simulink library "amg_high_precision_rtc"  (R2015b)
settings: Solver=ode45  StartTime=0.0  StopTime=10.0  RelTol=1e-3
libraries: simulink x207, waijung_soft_i2c_lib x11, amg_high_precision_rtc x10
(part 4 of 5)

== system amg_high_precision_rtc/Soft I2C/Soft-DS3231 Configure/Enabled Subsystem/Debouce2/Enabled Subsystem1 ==
  Enable : EnablePort  PropagateVarSize=During execution
  Bitwise Operator : simulink/Logic and Bit Operations/Bitwise Operator  logicop=AND  UseBitMask=on  BitMask=1  BitMaskRealWorld=Stored Integer
  Compare To Zero : simulink/Logic and Bit Operations/Compare To Zero  SystemSampleTime=-1  relop===  LogicOutDataTypeMode=uint8  ZeroCross=off
  Counter Free-Running : simulink/Sources/Counter Free-Running  SystemSampleTime=-1  NumBits=32  tsamp=-1
  Out1 : Outport  InitialOutput=0
  wires:
  Compare To Zero/1 -> Out1/1
  Bitwise Operator/1 -> Compare To Zero/1
  Counter Free-Running/1 -> Bitwise Operator/1

== system amg_high_precision_rtc/Soft I2C/Soft-DS3231 Configure/Enabled Subsystem/Debouce2/Enabled Subsystem4 ==
  Enable : EnablePort  PropagateVarSize=During execution
  Counter Free-Running : simulink/Sources/Counter Free-Running  SystemSampleTime=-1  NumBits=32  tsamp=-1
  Out1 : Outport  InitialOutput=0
  wires:
  Counter Free-Running/1 -> Out1/1

== system amg_high_precision_rtc/Soft I2C/Soft-DS3231 Configure/Enabled Subsystem/Debouce2/Enabled Subsystem5 ==
  Enable : EnablePort  PropagateVarSize=During execution
  Counter Free-Running : simulink/Sources/Counter Free-Running  SystemSampleTime=-1  NumBits=32  tsamp=-1
  Out1 : Outport  InitialOutput=0
  wires:
  Counter Free-Running/1 -> Out1/1

== system amg_high_precision_rtc/Soft I2C/Soft-DS3231 Configure/Enabled Subsystem/Debouce3/Enabled Subsystem ==
  Enable : EnablePort  PropagateVarSize=During execution
  Counter Free-Running : simulink/Sources/Counter Free-Running  SystemSampleTime=-1  NumBits=32  tsamp=-1
  Out1 : Outport  InitialOutput=0
  wires:
  Counter Free-Running/1 -> Out1/1

== system amg_high_precision_rtc/Soft I2C/Soft-DS3231 Configure/Enabled Subsystem/Debouce3/Enabled Subsystem1 ==
  Enable : EnablePort  PropagateVarSize=During execution
  Bitwise Operator : simulink/Logic and Bit Operations/Bitwise Operator  logicop=AND  UseBitMask=on  BitMask=1  BitMaskRealWorld=Stored Integer
  Compare To Zero : simulink/Logic and Bit Operations/Compare To Zero  SystemSampleTime=-1  relop===  LogicOutDataTypeMode=uint8  ZeroCross=off
  Counter Free-Running : simulink/Sources/Counter Free-Running  SystemSampleTime=-1  NumBits=32  tsamp=-1
  Out1 : Outport  InitialOutput=0
  wires:
  Compare To Zero/1 -> Out1/1
  Bitwise Operator/1 -> Compare To Zero/1
  Counter Free-Running/1 -> Bitwise Operator/1

== system amg_high_precision_rtc/Soft I2C/Soft-DS3231 Configure/Enabled Subsystem/Debouce3/Enabled Subsystem4 ==
  Enable : EnablePort  PropagateVarSize=During execution
  Counter Free-Running : simulink/Sources/Counter Free-Running  SystemSampleTime=-1  NumBits=32  tsamp=-1
  Out1 : Outport  InitialOutput=0
  wires:
  Counter Free-Running/1 -> Out1/1

== system amg_high_precision_rtc/Soft I2C/Soft-DS3231 Configure/Enabled Subsystem/Debouce3/Enabled Subsystem5 ==
  Enable : EnablePort  PropagateVarSize=During execution
  Counter Free-Running : simulink/Sources/Counter Free-Running  SystemSampleTime=-1  NumBits=32  tsamp=-1
  Out1 : Outport  InitialOutput=0
  wires:
  Counter Free-Running/1 -> Out1/1

== system amg_high_precision_rtc/Soft I2C/Soft-DS3231 Configure/Enabled Subsystem/Generate Mode ID/Enabled Subsystem2 ==
  Enable : EnablePort  PropagateVarSize=During execution
  Bitwise Operator : simulink/Logic and Bit Operations/Bitwise Operator  logicop=AND  UseBitMask=on  BitMask=7  BitMaskRealWorld=Stored Integer
  Counter Free-Running : simulink/Sources/Counter Free-Running  SystemSampleTime=-1  NumBits=16  tsamp=-1
  Out1 : Outport  InitialOutput=0
  wires:
  Bitwise Operator/1 -> Out1/1
  Counter Free-Running/1 -> Bitwise Operator/1

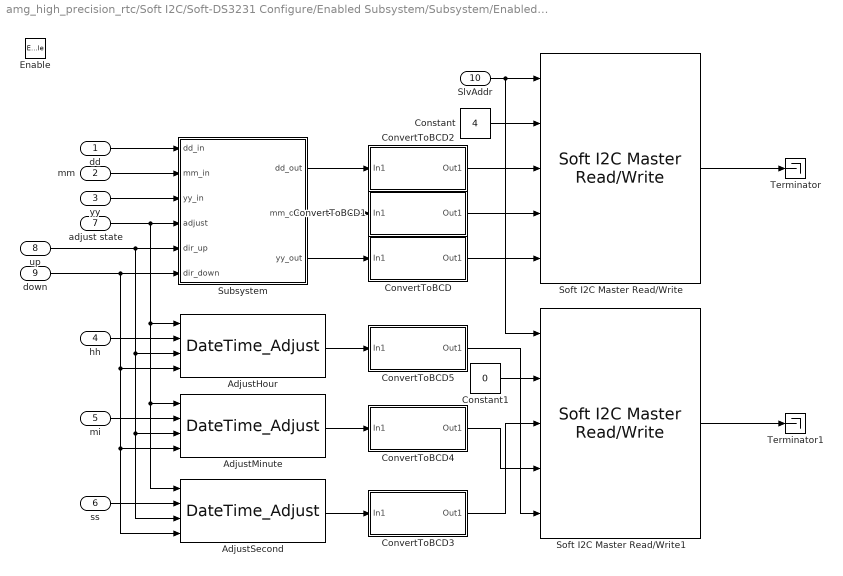
== system amg_high_precision_rtc/Soft I2C/Soft-DS3231 Configure/Enabled Subsystem/Subsystem/Enabled Subsystem ==
  dd : Inport
  mm : Inport  Port=2
  yy : Inport  Port=3
  hh : Inport  Port=4
  mi : Inport  Port=5
  ss : Inport  Port=6
  adjust state : Inport  Port=7
  up : Inport  Port=8
  down : Inport  Port=9
  SlvAddr : Inport  Port=10
  Enable : EnablePort  PropagateVarSize=During execution
  AdjustHour : amg_high_precision_rtc/DateTime_Adjust  SystemSampleTime=-1  state=3  max=23  min=0
  AdjustMinute : amg_high_precision_rtc/DateTime_Adjust  SystemSampleTime=-1  state=4  max=59  min=0
  AdjustSecond : amg_high_precision_rtc/DateTime_Adjust  SystemSampleTime=-1  state=5  max=59  min=0
  Constant : Constant  Value=4  OutDataTypeStr=uint8
  Constant1 : Constant  Value=0  OutDataTypeStr=uint8
  ConvertToBCD : Subsystem  TreatAsAtomicUnit=on
      settings: RTWFcnNameOpts=Use subsystem name  RTWFileNameOpts=Use function name
      mask Display: disp('Dec-to-BCD');
  ConvertToBCD1 : Subsystem  TreatAsAtomicUnit=on
      settings: RTWFcnNameOpts=Use subsystem name  RTWFileNameOpts=Use function name
      mask Display: disp('Dec-to-BCD');
  ConvertToBCD2 : Subsystem  TreatAsAtomicUnit=on
      settings: RTWFcnNameOpts=Use subsystem name  RTWFileNameOpts=Use function name
      mask Display: disp('Dec-to-BCD');
  ConvertToBCD3 : Subsystem  TreatAsAtomicUnit=on
      settings: RTWFcnNameOpts=Use subsystem name  RTWFileNameOpts=Use function name
      mask Display: disp('Dec-to-BCD');
  ConvertToBCD4 : Subsystem  TreatAsAtomicUnit=on
      settings: RTWFcnNameOpts=Use subsystem name  RTWFileNameOpts=Use function name
      mask Display: disp('Dec-to-BCD');
  ConvertToBCD5 : Subsystem  TreatAsAtomicUnit=on
      settings: RTWFcnNameOpts=Use subsystem name  RTWFileNameOpts=Use function name
      mask Display: disp('Dec-to-BCD');
  Soft I2C Master Read/Write : waijung_soft_i2c_lib/Soft I2C Master Read//Write  conf=ReadWrite  targetname=0  module=1  transfer=Blocking  clk=100  timeout=25  sdapins={'A4','A6'}  sclpins='A5'  writecount=4  readcount=0  waittime=0  forcestop=off  portpinstr=0  sampletime=inf  blockid=SoftI2CSoftDS3231ConfigureEnabledSubsystemSubsystemEnabledSubsystemSoftI2CMasterReadWrite  inputporttype=[3 3 3 3 3]  inputportwidth=[]  inputportlabel={'SlvAddr' 'Wr0 (uint8)' 'Wr1 (uint8)' 'Wr2 (uint8)' 'Wr3 (uint8)'}  outputporttype=[3]  outputportwidth=[1]  outputportlabel={'Status'}  compat=0  optionstring=[]
  Soft I2C Master Read/Write1 : waijung_soft_i2c_lib/Soft I2C Master Read//Write  conf=ReadWrite  targetname=0  module=1  transfer=Blocking  clk=100  timeout=25  sdapins={'A4','A6'}  sclpins='A5'  writecount=4  readcount=0  waittime=0  forcestop=off  portpinstr=0  sampletime=inf  blockid=SoftI2CSoftDS3231ConfigureEnabledSubsystemSubsystemEnabledSubsystemSoftI2CMasterReadWrite  inputporttype=[3 3 3 3 3]  inputportwidth=[]  inputportlabel={'SlvAddr' 'Wr0 (uint8)' 'Wr1 (uint8)' 'Wr2 (uint8)' 'Wr3 (uint8)'}  outputporttype=[3]  outputportwidth=[1]  outputportlabel={'Status'}  compat=0  optionstring=[]
  Subsystem : Subsystem
  Terminator : Terminator
  Terminator1 : Terminator
  wires:
  ConvertToBCD3/1(Out1) -> Soft I2C Master Read/Write1/3
  ConvertToBCD5/1(Out1) -> Soft I2C Master Read/Write1/5
  AdjustSecond/1 -> ConvertToBCD3/1(In1)
  AdjustMinute/1 -> ConvertToBCD4/1(In1)
  AdjustHour/1 -> ConvertToBCD5/1(In1)
  ConvertToBCD4/1(Out1) -> Soft I2C Master Read/Write1/4
  Soft I2C Master Read/Write1/1 -> Terminator1/1
  Constant1/1 -> Soft I2C Master Read/Write1/2
  hh/1 -> AdjustHour/2
  mi/1 -> AdjustMinute/2
  ss/1 -> AdjustSecond/2
  ConvertToBCD/1(Out1) -> Soft I2C Master Read/Write/5
  ConvertToBCD1/1(Out1) -> Soft I2C Master Read/Write/4
  ConvertToBCD2/1(Out1) -> Soft I2C Master Read/Write/3
  Soft I2C Master Read/Write/1 -> Terminator/1
  Constant/1 -> Soft I2C Master Read/Write/2
  Subsystem/3(yy_out) -> ConvertToBCD/1(In1)
  Subsystem/2(mm_out) -> ConvertToBCD1/1(In1)
  Subsystem/1(dd_out) -> ConvertToBCD2/1(In1)
  SlvAddr/1 -> Soft I2C Master Read/Write/1, Soft I2C Master Read/Write1/1
  down/1 -> AdjustSecond/4, AdjustMinute/4, AdjustHour/4, Subsystem/6(dir_down)
  up/1 -> AdjustSecond/3, AdjustMinute/3, AdjustHour/3, Subsystem/5(dir_up)
  adjust state/1 -> AdjustSecond/1, AdjustMinute/1, AdjustHour/1, Subsystem/4(adjust)
  yy/1 -> Subsystem/3(yy_in)
  mm/1 -> Subsystem/2(mm_in)
  dd/1 -> Subsystem/1(dd_in)

== system amg_high_precision_rtc/Soft I2C/Soft-DS3231 Configure/Enabled Subsystem/Subsystem/Soft-DS3231 Get Date ==
  Slave Address : Inport
  Compare To Zero : simulink/Logic and Bit Operations/Compare To Zero  SystemSampleTime=-1  relop===  LogicOutDataTypeMode=uint8  ZeroCross=off
  Convert : Subsystem  TreatAsAtomicUnit=on
  REG_DATE : Constant  Value=hex2dec('03')  OutDataTypeStr=uint8
  Soft I2C Master Read/Write : waijung_soft_i2c_lib/Soft I2C Master Read//Write  conf=ReadWrite  targetname=0  module=1  transfer=Blocking  clk=100  timeout=25  sdapins={'A4','A6'}  sclpins='A5'  writecount=1  readcount=4  waittime=0  forcestop=off  portpinstr=0  sampletime=-1  blockid=SoftI2CSoftDS3231GetDateSoftI2CMasterReadWrite  inputporttype=[3 3]  inputportwidth=[]  inputportlabel={'SlvAddr' 'Wr0 (uint8)'}  outputporttype="[3 3 3 3 3    ]"  outputportwidth=[1 1 1 1 1]  outputportlabel={'Status' 'Rd0 (uint8)' 'Rd1 (uint8)' 'Rd2 (uint8)' 'Rd3 (uint8)'}  compat=0  optionstring=[]
  Status : Outport
  Day : Outport  Port=2
  Date : Outport  Port=3
  Month : Outport  Port=4
  Year : Outport  Port=5
  wires:
  Soft I2C Master Read/Write/4 -> Convert/3(In3)
  Soft I2C Master Read/Write/3 -> Convert/2(In2)
  Soft I2C Master Read/Write/2 -> Convert/1(In1)
  Compare To Zero/1 -> Status/1, Convert/Enable
  Soft I2C Master Read/Write/1 -> Compare To Zero/1
  Slave Address/1 -> Soft I2C Master Read/Write/1
  REG_DATE/1 -> Soft I2C Master Read/Write/2
  Soft I2C Master Read/Write/5 -> Convert/4(In4)
  Convert/1(Day) -> Day/1
  Convert/2(Date) -> Date/1
  Convert/4(Year) -> Year/1
  Convert/3(Month) -> Month/1

== system amg_high_precision_rtc/Soft I2C/Soft-DS3231 Configure/Enabled Subsystem/Subsystem/Soft-DS3231 Get Time ==
  Slave Address : Inport
  Compare To Zero : simulink/Logic and Bit Operations/Compare To Zero  SystemSampleTime=-1  relop===  LogicOutDataTypeMode=uint8  ZeroCross=off
  Convert : Subsystem  TreatAsAtomicUnit=on
  Data Type Conversion{,1..3} (4 alike) : DataTypeConversion  OutDataTypeStr=uint8
  REG_TIME : Constant  Value=hex2dec('00')  OutDataTypeStr=uint8
  Soft I2C Master Read/Write : waijung_soft_i2c_lib/Soft I2C Master Read//Write  conf=ReadWrite  targetname=0  module=1  transfer=Blocking  clk=100  timeout=25  sdapins={'A4','A6'}  sclpins='A5'  writecount=1  readcount=3  waittime=0  forcestop=off  portpinstr=0  sampletime=-1  blockid=SoftI2CSoftDS3231GetTimeSoftI2CMasterReadWrite  inputporttype=[3 3]  inputportwidth=[]  inputportlabel={'SlvAddr' 'Wr0 (uint8)'}  outputporttype="[3 3 3 3   ]"  outputportwidth=[1 1 1 1]  outputportlabel={'Status' 'Rd0 (uint8)' 'Rd1 (uint8)' 'Rd2 (uint8)'}  compat=0  optionstring=[]
  Status : Outport
  Hour : Outport  Port=2
  Minute : Outport  Port=3
  Second : Outport  Port=4
  AM/PM : Outport  Port=5
  wires:
  REG_TIME/1 -> Soft I2C Master Read/Write/2
  Slave Address/1 -> Soft I2C Master Read/Write/1
  Soft I2C Master Read/Write/1 -> Compare To Zero/1
  Compare To Zero/1 -> Convert/Enable, Status/1
  Soft I2C Master Read/Write/2 -> Convert/1(In1)
  Soft I2C Master Read/Write/3 -> Convert/2(In2)
  Soft I2C Master Read/Write/4 -> Convert/3(In3)
  Convert/3(Second) -> Data Type Conversion2/1
  Convert/2(Minute) -> Data Type Conversion1/1
  Convert/1(Hour) -> Data Type Conversion/1
  Convert/4(AM/PM) -> Data Type Conversion3/1
  Data Type Conversion/1 -> Hour/1
  Data Type Conversion1/1 -> Minute/1
  Data Type Conversion2/1 -> Second/1
  Data Type Conversion3/1 -> AM/PM/1

== system amg_high_precision_rtc/STM32F4/DS3231 Configure/Enabled Subsystem/Subsystem/DS3231 Get Date/Convert ==
  In1 : Inport
  In2 : Inport  Port=2
  In3 : Inport  Port=3
  In4 : Inport  Port=4
  Enable : EnablePort  PropagateVarSize=During execution
  Convert 1 : Subsystem
  Convert 2 : Subsystem
  Convert 3 : Subsystem
  Data Type Conversion{,1..3} (4 alike) : DataTypeConversion  OutDataTypeStr=uint8
  Extract Bits : simulink/Logic and Bit Operations/Extract Bits  SystemSampleTime=-1  bitsToExtract=Range of bits  numBits=8  bitIdxRange=[0 3]  outScalingMode=Treat bit field as an integer
  Day : Outport
  Date : Outport  Port=2
  Month : Outport  Port=3
  Year : Outport  Port=4
  wires:
  Data Type Conversion3/1 -> Year/1
  Data Type Conversion2/1 -> Month/1
  Data Type Conversion1/1 -> Date/1
  Data Type Conversion/1 -> Day/1
  Convert 3/1(Out1) -> Data Type Conversion3/1
  In4/1 -> Convert 3/1(In1)
  Convert 2/1(Out1) -> Data Type Conversion2/1
  In3/1 -> Convert 2/1(In1)
  In2/1 -> Convert 1/1(In1)
  Convert 1/1(Out1) -> Data Type Conversion1/1
  Extract Bits/1 -> Data Type Conversion/1
  In1/1 -> Extract Bits/1

== system amg_high_precision_rtc/STM32F4/DS3231 Configure/Enabled Subsystem/Subsystem/DS3231 Get Time/Convert ==
  In1 : Inport
  In2 : Inport  Port=2
  In3 : Inport  Port=3
  Enable : EnablePort  PropagateVarSize=During execution
  Convert Hour : Subsystem
  Convert Second/ Minute : Subsystem
  Demux : Demux  Outputs=2
  Mux : Mux  Inputs=2
  Hour : Outport
  Minute : Outport  Port=2
  Second : Outport  Port=3
  AM/PM : Outport  Port=4
  wires:
  Convert Hour/2(AM/PM) -> AM/PM/1
  Convert Hour/1(Hour) -> Hour/1
  In3/1 -> Convert Hour/1(In1)
  Demux/2 -> Minute/1
  Demux/1 -> Second/1
  Convert Second/ Minute/1(Out1) -> Demux/1
  Mux/1 -> Convert Second/ Minute/1(In1)
  In1/1 -> Mux/1
  In2/1 -> Mux/2

== system amg_high_precision_rtc/STM32F4/DS3231 Configure/Enabled Subsystem/Subsystem/Enabled Subsystem/ConvertToBCD ==
  In1 : Inport
  Bitwise Operator : simulink/Logic and Bit Operations/Bitwise Operator  logicop=OR  UseBitMask=off  NumInputPorts=2  BitMask=bin2dec('11011001')  BitMaskRealWorld=Stored Integer
  Constant : Constant  Value=10  OutDataTypeStr=single
  Constant1 : Constant  Value=10  OutDataTypeStr=single
  Data Type Conversion : DataTypeConversion  OutDataTypeStr=single
  Data Type Conversion1 : DataTypeConversion  OutDataTypeStr=uint8
  Data Type Conversion2 : DataTypeConversion  OutDataTypeStr=uint8
  Data Type Conversion3 : DataTypeConversion  OutDataTypeStr=uint8
  Divide : Product  Inputs=*/
  Product : Product  RndMeth=Zero
  Shift Arithmetic : simulink/Logic and Bit Operations/Shift Arithmetic  SystemSampleTime=-1  nBitShiftRight=-4  nBinPtShiftRight=0
  Subtract : Sum  Inputs=+-
  Out1 : Outport
  wires:
  Bitwise Operator/1 -> Out1/1
  Data Type Conversion3/1 -> Bitwise Operator/2
  Data Type Conversion2/1 -> Bitwise Operator/1
  Shift Arithmetic/1 -> Data Type Conversion3/1
  Subtract/1 -> Data Type Conversion2/1
  Constant1/1 -> Product/1
  Product/1 -> Subtract/2
  Data Type Conversion1/1 -> Shift Arithmetic/1, Product/2
  Divide/1 -> Data Type Conversion1/1
  Data Type Conversion/1 -> Divide/1
  In1/1 -> Subtract/1, Data Type Conversion/1
  Constant/1 -> Divide/2

== system amg_high_precision_rtc/STM32F4/DS3231 Configure/Enabled Subsystem/Subsystem/Enabled Subsystem/ConvertToBCD1 ==
  In1 : Inport
  Bitwise Operator : simulink/Logic and Bit Operations/Bitwise Operator  logicop=OR  UseBitMask=off  NumInputPorts=2  BitMask=bin2dec('11011001')  BitMaskRealWorld=Stored Integer
  Constant : Constant  Value=10  OutDataTypeStr=single
  Constant1 : Constant  Value=10  OutDataTypeStr=single
  Data Type Conversion : DataTypeConversion  OutDataTypeStr=single
  Data Type Conversion1 : DataTypeConversion  OutDataTypeStr=uint8
  Data Type Conversion2 : DataTypeConversion  OutDataTypeStr=uint8
  Data Type Conversion3 : DataTypeConversion  OutDataTypeStr=uint8
  Divide : Product  Inputs=*/
  Product : Product  RndMeth=Zero
  Shift Arithmetic : simulink/Logic and Bit Operations/Shift Arithmetic  SystemSampleTime=-1  nBitShiftRight=-4  nBinPtShiftRight=0
  Subtract : Sum  Inputs=+-
  Out1 : Outport
  wires:
  Bitwise Operator/1 -> Out1/1
  Data Type Conversion3/1 -> Bitwise Operator/2
  Data Type Conversion2/1 -> Bitwise Operator/1
  Shift Arithmetic/1 -> Data Type Conversion3/1
  Subtract/1 -> Data Type Conversion2/1
  Constant1/1 -> Product/1
  Product/1 -> Subtract/2
  Data Type Conversion1/1 -> Shift Arithmetic/1, Product/2
  Divide/1 -> Data Type Conversion1/1
  Data Type Conversion/1 -> Divide/1
  In1/1 -> Subtract/1, Data Type Conversion/1
  Constant/1 -> Divide/2

== system amg_high_precision_rtc/STM32F4/DS3231 Configure/Enabled Subsystem/Subsystem/Enabled Subsystem/ConvertToBCD2 ==
  In1 : Inport
  Bitwise Operator : simulink/Logic and Bit Operations/Bitwise Operator  logicop=OR  UseBitMask=off  NumInputPorts=2  BitMask=bin2dec('11011001')  BitMaskRealWorld=Stored Integer
  Constant : Constant  Value=10  OutDataTypeStr=single
  Constant1 : Constant  Value=10  OutDataTypeStr=single
  Data Type Conversion : DataTypeConversion  OutDataTypeStr=single
  Data Type Conversion1 : DataTypeConversion  OutDataTypeStr=uint8
  Data Type Conversion2 : DataTypeConversion  OutDataTypeStr=uint8
  Data Type Conversion3 : DataTypeConversion  OutDataTypeStr=uint8
  Divide : Product  Inputs=*/
  Product : Product  RndMeth=Zero
  Shift Arithmetic : simulink/Logic and Bit Operations/Shift Arithmetic  SystemSampleTime=-1  nBitShiftRight=-4  nBinPtShiftRight=0
  Subtract : Sum  Inputs=+-
  Out1 : Outport
  wires:
  Bitwise Operator/1 -> Out1/1
  Data Type Conversion3/1 -> Bitwise Operator/2
  Data Type Conversion2/1 -> Bitwise Operator/1
  Shift Arithmetic/1 -> Data Type Conversion3/1
  Subtract/1 -> Data Type Conversion2/1
  Constant1/1 -> Product/1
  Product/1 -> Subtract/2
  Data Type Conversion1/1 -> Shift Arithmetic/1, Product/2
  Divide/1 -> Data Type Conversion1/1
  Data Type Conversion/1 -> Divide/1
  In1/1 -> Subtract/1, Data Type Conversion/1
  Constant/1 -> Divide/2

== system amg_high_precision_rtc/STM32F4/DS3231 Configure/Enabled Subsystem/Subsystem/Enabled Subsystem/ConvertToBCD3 ==
  In1 : Inport
  Bitwise Operator : simulink/Logic and Bit Operations/Bitwise Operator  logicop=OR  UseBitMask=off  NumInputPorts=2  BitMask=bin2dec('11011001')  BitMaskRealWorld=Stored Integer
  Constant : Constant  Value=10  OutDataTypeStr=single
  Constant1 : Constant  Value=10  OutDataTypeStr=single
  Data Type Conversion : DataTypeConversion  OutDataTypeStr=single
  Data Type Conversion1 : DataTypeConversion  OutDataTypeStr=uint8
  Data Type Conversion2 : DataTypeConversion  OutDataTypeStr=uint8
  Data Type Conversion3 : DataTypeConversion  OutDataTypeStr=uint8
  Divide : Product  Inputs=*/
  Product : Product  RndMeth=Zero
  Shift Arithmetic : simulink/Logic and Bit Operations/Shift Arithmetic  SystemSampleTime=-1  nBitShiftRight=-4  nBinPtShiftRight=0
  Subtract : Sum  Inputs=+-
  Out1 : Outport
  wires:
  Bitwise Operator/1 -> Out1/1
  Data Type Conversion3/1 -> Bitwise Operator/2
  Data Type Conversion2/1 -> Bitwise Operator/1
  Shift Arithmetic/1 -> Data Type Conversion3/1
  Subtract/1 -> Data Type Conversion2/1
  Constant1/1 -> Product/1
  Product/1 -> Subtract/2
  Data Type Conversion1/1 -> Shift Arithmetic/1, Product/2
  Divide/1 -> Data Type Conversion1/1
  Data Type Conversion/1 -> Divide/1
  In1/1 -> Subtract/1, Data Type Conversion/1
  Constant/1 -> Divide/2

== system amg_high_precision_rtc/STM32F4/DS3231 Configure/Enabled Subsystem/Subsystem/Enabled Subsystem/ConvertToBCD4 ==
  In1 : Inport
  Bitwise Operator : simulink/Logic and Bit Operations/Bitwise Operator  logicop=OR  UseBitMask=off  NumInputPorts=2  BitMask=bin2dec('11011001')  BitMaskRealWorld=Stored Integer
  Constant : Constant  Value=10  OutDataTypeStr=single
  Constant1 : Constant  Value=10  OutDataTypeStr=single
  Data Type Conversion : DataTypeConversion  OutDataTypeStr=single
  Data Type Conversion1 : DataTypeConversion  OutDataTypeStr=uint8
  Data Type Conversion2 : DataTypeConversion  OutDataTypeStr=uint8
  Data Type Conversion3 : DataTypeConversion  OutDataTypeStr=uint8
  Divide : Product  Inputs=*/
  Product : Product  RndMeth=Zero
  Shift Arithmetic : simulink/Logic and Bit Operations/Shift Arithmetic  SystemSampleTime=-1  nBitShiftRight=-4  nBinPtShiftRight=0
  Subtract : Sum  Inputs=+-
  Out1 : Outport
  wires:
  Bitwise Operator/1 -> Out1/1
  Data Type Conversion3/1 -> Bitwise Operator/2
  Data Type Conversion2/1 -> Bitwise Operator/1
  Shift Arithmetic/1 -> Data Type Conversion3/1
  Subtract/1 -> Data Type Conversion2/1
  Constant1/1 -> Product/1
  Product/1 -> Subtract/2
  Data Type Conversion1/1 -> Shift Arithmetic/1, Product/2
  Divide/1 -> Data Type Conversion1/1
  Data Type Conversion/1 -> Divide/1
  In1/1 -> Subtract/1, Data Type Conversion/1
  Constant/1 -> Divide/2

== system amg_high_precision_rtc/STM32F4/DS3231 Configure/Enabled Subsystem/Subsystem/Enabled Subsystem/ConvertToBCD5 ==
  In1 : Inport
  Bitwise Operator : simulink/Logic and Bit Operations/Bitwise Operator  logicop=OR  UseBitMask=off  NumInputPorts=2  BitMask=bin2dec('11011001')  BitMaskRealWorld=Stored Integer
  Constant : Constant  Value=10  OutDataTypeStr=single
  Constant1 : Constant  Value=10  OutDataTypeStr=single
  Data Type Conversion : DataTypeConversion  OutDataTypeStr=single
  Data Type Conversion1 : DataTypeConversion  OutDataTypeStr=uint8
  Data Type Conversion2 : DataTypeConversion  OutDataTypeStr=uint8
  Data Type Conversion3 : DataTypeConversion  OutDataTypeStr=uint8
  Divide : Product  Inputs=*/
  Product : Product  RndMeth=Zero
  Shift Arithmetic : simulink/Logic and Bit Operations/Shift Arithmetic  SystemSampleTime=-1  nBitShiftRight=-4  nBinPtShiftRight=0
  Subtract : Sum  Inputs=+-
  Out1 : Outport
  wires:
  Bitwise Operator/1 -> Out1/1
  Data Type Conversion3/1 -> Bitwise Operator/2
  Data Type Conversion2/1 -> Bitwise Operator/1
  Shift Arithmetic/1 -> Data Type Conversion3/1
  Subtract/1 -> Data Type Conversion2/1
  Constant1/1 -> Product/1
  Product/1 -> Subtract/2
  Data Type Conversion1/1 -> Shift Arithmetic/1, Product/2
  Divide/1 -> Data Type Conversion1/1
  Data Type Conversion/1 -> Divide/1
  In1/1 -> Subtract/1, Data Type Conversion/1
  Constant/1 -> Divide/2

== system amg_high_precision_rtc/STM32F4/DS3231 Configure/Enabled Subsystem/Subsystem/Enabled Subsystem/Subsystem ==
  dd_in : Inport
  mm_in : Inport  Port=2
  yy_in : Inport  Port=3
  adjust : Inport  Port=4
  dir_up : Inport  Port=5
  dir_down : Inport  Port=6
  AdjustMonth : amg_high_precision_rtc/DateTime_Adjust  SystemSampleTime=-1  state=1  max=12  min=1
  AdjustYear : amg_high_precision_rtc/DateTime_Adjust  SystemSampleTime=-1  state=2  max=99  min=0
  Day count : Subsystem
  Relational Operator : RelationalOperator  Operator=>  OutDataTypeStr=boolean
  Subsystem : Subsystem
  Switch : Switch  Criteria=u2 ~= 0
  dd_out : Outport
  mm_out : Outport  Port=2
  yy_out : Outport  Port=3
  wires:
  dir_down/1 -> AdjustYear/4, AdjustMonth/4, Subsystem/4(Down)
  dir_up/1 -> AdjustYear/3, AdjustMonth/3, Subsystem/3(Up)
  adjust/1 -> AdjustYear/1, AdjustMonth/1, Subsystem/1(Function)
  yy_in/1 -> AdjustYear/2
  mm_in/1 -> AdjustMonth/2
  AdjustYear/1 -> Day count/2(Year), yy_out/1
  AdjustMonth/1 -> Day count/1(Month), mm_out/1
  dd_in/1 -> Relational Operator/1, Switch/3
  Switch/1 -> Subsystem/2(Input)
  Day count/1(Day count of month) -> Relational Operator/2, Switch/1, Subsystem/5(Day count)
  Relational Operator/1 -> Switch/2
  Subsystem/1(Output) -> dd_out/1

== system amg_high_precision_rtc/Soft I2C/Soft-DS3231 Configure/Enabled Subsystem/Subsystem/Enabled Subsystem/ConvertToBCD ==
  In1 : Inport
  Bitwise Operator : simulink/Logic and Bit Operations/Bitwise Operator  logicop=OR  UseBitMask=off  NumInputPorts=2  BitMask=bin2dec('11011001')  BitMaskRealWorld=Stored Integer
  Constant : Constant  Value=10  OutDataTypeStr=single
  Constant1 : Constant  Value=10  OutDataTypeStr=single
  Data Type Conversion : DataTypeConversion  OutDataTypeStr=single
  Data Type Conversion1 : DataTypeConversion  OutDataTypeStr=uint8
  Data Type Conversion2 : DataTypeConversion  OutDataTypeStr=uint8
  Data Type Conversion3 : DataTypeConversion  OutDataTypeStr=uint8
  Divide : Product  Inputs=*/
  Product : Product  RndMeth=Zero
  Shift Arithmetic : simulink/Logic and Bit Operations/Shift Arithmetic  SystemSampleTime=-1  nBitShiftRight=-4  nBinPtShiftRight=0
  Subtract : Sum  Inputs=+-
  Out1 : Outport
  wires:
  Constant/1 -> Divide/2
  In1/1 -> Data Type Conversion/1, Subtract/1
  Data Type Conversion/1 -> Divide/1
  Divide/1 -> Data Type Conversion1/1
  Data Type Conversion1/1 -> Product/2, Shift Arithmetic/1
  Product/1 -> Subtract/2
  Constant1/1 -> Product/1
  Subtract/1 -> Data Type Conversion2/1
  Shift Arithmetic/1 -> Data Type Conversion3/1
  Data Type Conversion2/1 -> Bitwise Operator/1
  Data Type Conversion3/1 -> Bitwise Operator/2
  Bitwise Operator/1 -> Out1/1

== system amg_high_precision_rtc/Soft I2C/Soft-DS3231 Configure/Enabled Subsystem/Subsystem/Enabled Subsystem/ConvertToBCD1 ==
  In1 : Inport
  Bitwise Operator : simulink/Logic and Bit Operations/Bitwise Operator  logicop=OR  UseBitMask=off  NumInputPorts=2  BitMask=bin2dec('11011001')  BitMaskRealWorld=Stored Integer
  Constant : Constant  Value=10  OutDataTypeStr=single
  Constant1 : Constant  Value=10  OutDataTypeStr=single
  Data Type Conversion : DataTypeConversion  OutDataTypeStr=single
  Data Type Conversion1 : DataTypeConversion  OutDataTypeStr=uint8
  Data Type Conversion2 : DataTypeConversion  OutDataTypeStr=uint8
  Data Type Conversion3 : DataTypeConversion  OutDataTypeStr=uint8
  Divide : Product  Inputs=*/
  Product : Product  RndMeth=Zero
  Shift Arithmetic : simulink/Logic and Bit Operations/Shift Arithmetic  SystemSampleTime=-1  nBitShiftRight=-4  nBinPtShiftRight=0
  Subtract : Sum  Inputs=+-
  Out1 : Outport
  wires:
  Constant/1 -> Divide/2
  In1/1 -> Data Type Conversion/1, Subtract/1
  Data Type Conversion/1 -> Divide/1
  Divide/1 -> Data Type Conversion1/1
  Data Type Conversion1/1 -> Product/2, Shift Arithmetic/1
  Product/1 -> Subtract/2
  Constant1/1 -> Product/1
  Subtract/1 -> Data Type Conversion2/1
  Shift Arithmetic/1 -> Data Type Conversion3/1
  Data Type Conversion2/1 -> Bitwise Operator/1
  Data Type Conversion3/1 -> Bitwise Operator/2
  Bitwise Operator/1 -> Out1/1

== system amg_high_precision_rtc/Soft I2C/Soft-DS3231 Configure/Enabled Subsystem/Subsystem/Enabled Subsystem/ConvertToBCD2 ==
  In1 : Inport
  Bitwise Operator : simulink/Logic and Bit Operations/Bitwise Operator  logicop=OR  UseBitMask=off  NumInputPorts=2  BitMask=bin2dec('11011001')  BitMaskRealWorld=Stored Integer
  Constant : Constant  Value=10  OutDataTypeStr=single
  Constant1 : Constant  Value=10  OutDataTypeStr=single
  Data Type Conversion : DataTypeConversion  OutDataTypeStr=single
  Data Type Conversion1 : DataTypeConversion  OutDataTypeStr=uint8
  Data Type Conversion2 : DataTypeConversion  OutDataTypeStr=uint8
  Data Type Conversion3 : DataTypeConversion  OutDataTypeStr=uint8
  Divide : Product  Inputs=*/
  Product : Product  RndMeth=Zero
  Shift Arithmetic : simulink/Logic and Bit Operations/Shift Arithmetic  SystemSampleTime=-1  nBitShiftRight=-4  nBinPtShiftRight=0
  Subtract : Sum  Inputs=+-
  Out1 : Outport
  wires:
  Constant/1 -> Divide/2
  In1/1 -> Data Type Conversion/1, Subtract/1
  Data Type Conversion/1 -> Divide/1
  Divide/1 -> Data Type Conversion1/1
  Data Type Conversion1/1 -> Product/2, Shift Arithmetic/1
  Product/1 -> Subtract/2
  Constant1/1 -> Product/1
  Subtract/1 -> Data Type Conversion2/1
  Shift Arithmetic/1 -> Data Type Conversion3/1
  Data Type Conversion2/1 -> Bitwise Operator/1
  Data Type Conversion3/1 -> Bitwise Operator/2
  Bitwise Operator/1 -> Out1/1

== system amg_high_precision_rtc/Soft I2C/Soft-DS3231 Configure/Enabled Subsystem/Subsystem/Enabled Subsystem/ConvertToBCD3 ==
  In1 : Inport
  Bitwise Operator : simulink/Logic and Bit Operations/Bitwise Operator  logicop=OR  UseBitMask=off  NumInputPorts=2  BitMask=bin2dec('11011001')  BitMaskRealWorld=Stored Integer
  Constant : Constant  Value=10  OutDataTypeStr=single
  Constant1 : Constant  Value=10  OutDataTypeStr=single
  Data Type Conversion : DataTypeConversion  OutDataTypeStr=single
  Data Type Conversion1 : DataTypeConversion  OutDataTypeStr=uint8
  Data Type Conversion2 : DataTypeConversion  OutDataTypeStr=uint8
  Data Type Conversion3 : DataTypeConversion  OutDataTypeStr=uint8
  Divide : Product  Inputs=*/
  Product : Product  RndMeth=Zero
  Shift Arithmetic : simulink/Logic and Bit Operations/Shift Arithmetic  SystemSampleTime=-1  nBitShiftRight=-4  nBinPtShiftRight=0
  Subtract : Sum  Inputs=+-
  Out1 : Outport
  wires:
  Constant/1 -> Divide/2
  In1/1 -> Data Type Conversion/1, Subtract/1
  Data Type Conversion/1 -> Divide/1
  Divide/1 -> Data Type Conversion1/1
  Data Type Conversion1/1 -> Product/2, Shift Arithmetic/1
  Product/1 -> Subtract/2
  Constant1/1 -> Product/1
  Subtract/1 -> Data Type Conversion2/1
  Shift Arithmetic/1 -> Data Type Conversion3/1
  Data Type Conversion2/1 -> Bitwise Operator/1
  Data Type Conversion3/1 -> Bitwise Operator/2
  Bitwise Operator/1 -> Out1/1

== system amg_high_precision_rtc/Soft I2C/Soft-DS3231 Configure/Enabled Subsystem/Subsystem/Enabled Subsystem/ConvertToBCD4 ==
  In1 : Inport
  Bitwise Operator : simulink/Logic and Bit Operations/Bitwise Operator  logicop=OR  UseBitMask=off  NumInputPorts=2  BitMask=bin2dec('11011001')  BitMaskRealWorld=Stored Integer
  Constant : Constant  Value=10  OutDataTypeStr=single
  Constant1 : Constant  Value=10  OutDataTypeStr=single
  Data Type Conversion : DataTypeConversion  OutDataTypeStr=single
  Data Type Conversion1 : DataTypeConversion  OutDataTypeStr=uint8
  Data Type Conversion2 : DataTypeConversion  OutDataTypeStr=uint8
  Data Type Conversion3 : DataTypeConversion  OutDataTypeStr=uint8
  Divide : Product  Inputs=*/
  Product : Product  RndMeth=Zero
  Shift Arithmetic : simulink/Logic and Bit Operations/Shift Arithmetic  SystemSampleTime=-1  nBitShiftRight=-4  nBinPtShiftRight=0
  Subtract : Sum  Inputs=+-
  Out1 : Outport
  wires:
  Constant/1 -> Divide/2
  In1/1 -> Data Type Conversion/1, Subtract/1
  Data Type Conversion/1 -> Divide/1
  Divide/1 -> Data Type Conversion1/1
  Data Type Conversion1/1 -> Product/2, Shift Arithmetic/1
  Product/1 -> Subtract/2
  Constant1/1 -> Product/1
  Subtract/1 -> Data Type Conversion2/1
  Shift Arithmetic/1 -> Data Type Conversion3/1
  Data Type Conversion2/1 -> Bitwise Operator/1
  Data Type Conversion3/1 -> Bitwise Operator/2
  Bitwise Operator/1 -> Out1/1

== system amg_high_precision_rtc/Soft I2C/Soft-DS3231 Configure/Enabled Subsystem/Subsystem/Enabled Subsystem/ConvertToBCD5 ==
  In1 : Inport
  Bitwise Operator : simulink/Logic and Bit Operations/Bitwise Operator  logicop=OR  UseBitMask=off  NumInputPorts=2  BitMask=bin2dec('11011001')  BitMaskRealWorld=Stored Integer
  Constant : Constant  Value=10  OutDataTypeStr=single
  Constant1 : Constant  Value=10  OutDataTypeStr=single
  Data Type Conversion : DataTypeConversion  OutDataTypeStr=single
  Data Type Conversion1 : DataTypeConversion  OutDataTypeStr=uint8
  Data Type Conversion2 : DataTypeConversion  OutDataTypeStr=uint8
  Data Type Conversion3 : DataTypeConversion  OutDataTypeStr=uint8
  Divide : Product  Inputs=*/
  Product : Product  RndMeth=Zero
  Shift Arithmetic : simulink/Logic and Bit Operations/Shift Arithmetic  SystemSampleTime=-1  nBitShiftRight=-4  nBinPtShiftRight=0
  Subtract : Sum  Inputs=+-
  Out1 : Outport
  wires:
  Constant/1 -> Divide/2
  In1/1 -> Data Type Conversion/1, Subtract/1
  Data Type Conversion/1 -> Divide/1
  Divide/1 -> Data Type Conversion1/1
  Data Type Conversion1/1 -> Product/2, Shift Arithmetic/1
  Product/1 -> Subtract/2
  Constant1/1 -> Product/1
  Subtract/1 -> Data Type Conversion2/1
  Shift Arithmetic/1 -> Data Type Conversion3/1
  Data Type Conversion2/1 -> Bitwise Operator/1
  Data Type Conversion3/1 -> Bitwise Operator/2
  Bitwise Operator/1 -> Out1/1

== system amg_high_precision_rtc/Soft I2C/Soft-DS3231 Configure/Enabled Subsystem/Subsystem/Enabled Subsystem/Subsystem ==
  dd_in : Inport
  mm_in : Inport  Port=2
  yy_in : Inport  Port=3
  adjust : Inport  Port=4
  dir_up : Inport  Port=5
  dir_down : Inport  Port=6
  AdjustMonth : amg_high_precision_rtc/DateTime_Adjust  SystemSampleTime=-1  state=1  max=12  min=1
  AdjustYear : amg_high_precision_rtc/DateTime_Adjust  SystemSampleTime=-1  state=2  max=99  min=0
  Day count : Subsystem
  Relational Operator : RelationalOperator  Operator=>  OutDataTypeStr=boolean
  Subsystem : Subsystem
  Switch : Switch  Criteria=u2 ~= 0
  dd_out : Outport
  mm_out : Outport  Port=2
  yy_out : Outport  Port=3
  wires:
  Subsystem/1(Output) -> dd_out/1
  Relational Operator/1 -> Switch/2
  Day count/1(Day count of month) -> Subsystem/5(Day count), Switch/1, Relational Operator/2
  Switch/1 -> Subsystem/2(Input)
  dd_in/1 -> Switch/3, Relational Operator/1
  AdjustMonth/1 -> mm_out/1, Day count/1(Month)
  AdjustYear/1 -> yy_out/1, Day count/2(Year)
  mm_in/1 -> AdjustMonth/2
  yy_in/1 -> AdjustYear/2
  adjust/1 -> Subsystem/1(Function), AdjustMonth/1, AdjustYear/1
  dir_up/1 -> Subsystem/3(Up), AdjustMonth/3, AdjustYear/3
  dir_down/1 -> Subsystem/4(Down), AdjustMonth/4, AdjustYear/4

== system amg_high_precision_rtc/Soft I2C/Soft-DS3231 Configure/Enabled Subsystem/Subsystem/Soft-DS3231 Get Date/Convert ==
  In1 : Inport
  In2 : Inport  Port=2
  In3 : Inport  Port=3
  In4 : Inport  Port=4
  Enable : EnablePort  PropagateVarSize=During execution
  Convert 1 : Subsystem
  Convert 2 : Subsystem
  Convert 3 : Subsystem
  Data Type Conversion{,1..3} (4 alike) : DataTypeConversion  OutDataTypeStr=uint8
  Extract Bits : simulink/Logic and Bit Operations/Extract Bits  SystemSampleTime=-1  bitsToExtract=Range of bits  numBits=8  bitIdxRange=[0 3]  outScalingMode=Treat bit field as an integer
  Day : Outport
  Date : Outport  Port=2
  Month : Outport  Port=3
  Year : Outport  Port=4
  wires:
  In1/1 -> Extract Bits/1
  Extract Bits/1 -> Data Type Conversion/1
  Convert 1/1(Out1) -> Data Type Conversion1/1
  In2/1 -> Convert 1/1(In1)
  In3/1 -> Convert 2/1(In1)
  Convert 2/1(Out1) -> Data Type Conversion2/1
  In4/1 -> Convert 3/1(In1)
  Convert 3/1(Out1) -> Data Type Conversion3/1
  Data Type Conversion/1 -> Day/1
  Data Type Conversion1/1 -> Date/1
  Data Type Conversion2/1 -> Month/1
  Data Type Conversion3/1 -> Year/1

== system amg_high_precision_rtc/Soft I2C/Soft-DS3231 Configure/Enabled Subsystem/Subsystem/Soft-DS3231 Get Time/Convert ==
  In1 : Inport
  In2 : Inport  Port=2
  In3 : Inport  Port=3
  Enable : EnablePort  PropagateVarSize=During execution
  Convert Hour : Subsystem
  Convert Second/ Minute : Subsystem
  Demux : Demux  Outputs=2
  Mux : Mux  Inputs=2
  Hour : Outport
  Minute : Outport  Port=2
  Second : Outport  Port=3
  AM/PM : Outport  Port=4
  wires:
  In2/1 -> Mux/2
  In1/1 -> Mux/1
  Mux/1 -> Convert Second/ Minute/1(In1)
  Convert Second/ Minute/1(Out1) -> Demux/1
  Demux/1 -> Second/1
  Demux/2 -> Minute/1
  In3/1 -> Convert Hour/1(In1)
  Convert Hour/1(Hour) -> Hour/1
  Convert Hour/2(AM/PM) -> AM/PM/1

== system amg_high_precision_rtc/STM32F4/DS3231 Configure/Enabled Subsystem/Subsystem/DS3231 Get Date/Convert/Convert 1 ==
  In1 : Inport
  Add : Sum
  Constant : Constant  Value=10  OutDataTypeStr=uint8
  Extract Bits : simulink/Logic and Bit Operations/Extract Bits  SystemSampleTime=-1  bitsToExtract=Range of bits  numBits=8  bitIdxRange=[4 5]  outScalingMode=Treat bit field as an integer
  Extract Bits1 : simulink/Logic and Bit Operations/Extract Bits  SystemSampleTime=-1  bitsToExtract=Range of bits  numBits=8  bitIdxRange=[0 3]  outScalingMode=Treat bit field as an integer
  Product : Product  RndMeth=Zero
  Out1 : Outport
  wires:
  Add/1 -> Out1/1
  Extract Bits1/1 -> Add/2
  Product/1 -> Add/1
  Extract Bits/1 -> Product/2
  Constant/1 -> Product/1
  In1/1 -> Extract Bits1/1, Extract Bits/1

== system amg_high_precision_rtc/STM32F4/DS3231 Configure/Enabled Subsystem/Subsystem/DS3231 Get Date/Convert/Convert 2 ==
  In1 : Inport
  Add : Sum
  Constant : Constant  Value=10  OutDataTypeStr=uint8
  Extract Bits : simulink/Logic and Bit Operations/Extract Bits  SystemSampleTime=-1  bitsToExtract=Range of bits  numBits=8  bitIdxRange=[4 4]  outScalingMode=Treat bit field as an integer
  Extract Bits1 : simulink/Logic and Bit Operations/Extract Bits  SystemSampleTime=-1  bitsToExtract=Range of bits  numBits=8  bitIdxRange=[0 3]  outScalingMode=Treat bit field as an integer
  Product : Product  RndMeth=Zero
  Out1 : Outport
  wires:
  In1/1 -> Extract Bits/1, Extract Bits1/1
  Constant/1 -> Product/1
  Extract Bits/1 -> Product/2
  Product/1 -> Add/1
  Extract Bits1/1 -> Add/2
  Add/1 -> Out1/1

== system amg_high_precision_rtc/STM32F4/DS3231 Configure/Enabled Subsystem/Subsystem/DS3231 Get Date/Convert/Convert 3 ==
  In1 : Inport
  Add : Sum
  Constant : Constant  Value=10  OutDataTypeStr=uint8
  Extract Bits : simulink/Logic and Bit Operations/Extract Bits  SystemSampleTime=-1  bitsToExtract=Range of bits  numBits=8  bitIdxRange=[4 7]  outScalingMode=Treat bit field as an integer
  Extract Bits1 : simulink/Logic and Bit Operations/Extract Bits  SystemSampleTime=-1  bitsToExtract=Range of bits  numBits=8  bitIdxRange=[0 3]  outScalingMode=Treat bit field as an integer
  Product : Product  RndMeth=Zero
  Out1 : Outport
  wires:
  Add/1 -> Out1/1
  Extract Bits1/1 -> Add/2
  Product/1 -> Add/1
  Extract Bits/1 -> Product/2
  Constant/1 -> Product/1
  In1/1 -> Extract Bits1/1, Extract Bits/1

== system amg_high_precision_rtc/STM32F4/DS3231 Configure/Enabled Subsystem/Subsystem/DS3231 Get Time/Convert/Convert Hour ==
  In1 : Inport
  Add : Sum
  Constant : Constant  Value=10  OutDataTypeStr=uint8
  Extract Bits : simulink/Logic and Bit Operations/Extract Bits  SystemSampleTime=-1  bitsToExtract=Range of bits  numBits=8  bitIdxRange=[4 5]  outScalingMode=Treat bit field as an integer
  Extract Bits1 : simulink/Logic and Bit Operations/Extract Bits  SystemSampleTime=-1  bitsToExtract=Range of bits  numBits=8  bitIdxRange=[0 3]  outScalingMode=Treat bit field as an integer
  Extract Bits2 : simulink/Logic and Bit Operations/Extract Bits  SystemSampleTime=-1  bitsToExtract=Range of bits  numBits=8  bitIdxRange=[5 5]  outScalingMode=Treat bit field as an integer
  Product : Product  RndMeth=Zero
  Hour : Outport
  AM/PM : Outport  Port=2
  wires:
  Extract Bits2/1 -> AM/PM/1
  Extract Bits1/1 -> Add/2
  In1/1 -> Extract Bits2/1, Extract Bits1/1, Extract Bits/1
  Constant/1 -> Product/1
  Extract Bits/1 -> Product/2
  Product/1 -> Add/1
  Add/1 -> Hour/1

== system amg_high_precision_rtc/STM32F4/DS3231 Configure/Enabled Subsystem/Subsystem/DS3231 Get Time/Convert/Convert Second// Minute ==
  In1 : Inport
  Add : Sum
  Constant : Constant  Value=10  OutDataTypeStr=uint8
  Extract Bits : simulink/Logic and Bit Operations/Extract Bits  SystemSampleTime=-1  bitsToExtract=Range of bits  numBits=8  bitIdxRange=[4 6]  outScalingMode=Treat bit field as an integer
  Extract Bits1 : simulink/Logic and Bit Operations/Extract Bits  SystemSampleTime=-1  bitsToExtract=Range of bits  numBits=8  bitIdxRange=[0 3]  outScalingMode=Treat bit field as an integer
  Product : Product  RndMeth=Zero
  Out1 : Outport
  wires:
  Add/1 -> Out1/1
  Extract Bits1/1 -> Add/2
  Product/1 -> Add/1
  Extract Bits/1 -> Product/2
  Constant/1 -> Product/1
  In1/1 -> Extract Bits1/1, Extract Bits/1

== system amg_high_precision_rtc/STM32F4/DS3231 Configure/Enabled Subsystem/Subsystem/Enabled Subsystem/Subsystem/Day count ==
  Month : Inport
  Year : Inport  Port=2
  Constant : Constant  Value=30  OutDataTypeStr=uint8
  Constant1 : Constant  Value=31  OutDataTypeStr=uint8
  Days 30 : Subsystem
  Subsystem : Subsystem
  Switch : Switch  Criteria=u2 ~= 0
  Switch1 : Switch  Criteria=u2 ~= 0
  Day count of month : Outport
  wires:
  Days 30/1(Out1) -> Switch/2
  Constant/1 -> Switch/1
  Month/1 -> Days 30/1(In1), Subsystem/1(Month)
  Year/1 -> Subsystem/2(Year)
  Subsystem/1(Out1) -> Switch1/2
  Subsystem/2(Day count) -> Switch1/1
  Constant1/1 -> Switch1/3
  Switch1/1 -> Switch/3
  Switch/1 -> Day count of month/1

== system amg_high_precision_rtc/STM32F4/DS3231 Configure/Enabled Subsystem/Subsystem/Enabled Subsystem/Subsystem/Subsystem ==
  Function : Inport
  Input : Inport  Port=2
  Up : Inport  Port=3
  Down : Inport  Port=4
  Day count : Inport  Port=5
  Compare To Constant : simulink/Logic and Bit Operations/Compare To Constant  SystemSampleTime=-1  relop===  const=0  LogicOutDataTypeMode=uint8  ZeroCross=off
  Constant : Constant  OutDataTypeStr=uint8
  Constant2 : Constant  OutDataTypeStr=uint8
  Min : Constant  OutDataTypeStr=uint8
  Relational Operator : RelationalOperator  Operator=<  OutDataTypeStr=boolean
  Relational Operator1 : RelationalOperator  Operator=>  OutDataTypeStr=boolean
  Subtract : Sum  Inputs=+-
  Subtract1 : Sum
  Switch{,1..4} (5 alike) : Switch  Criteria=u2 ~= 0
  Output : Outport
  wires:
  Switch1/1 -> Switch/3
  Input/1 -> Subtract/1, Switch1/3, Relational Operator1/1, Relational Operator/1, Subtract1/1, Switch4/3
  Relational Operator1/1 -> Switch2/2
  Subtract/1 -> Switch2/1
  Constant/1 -> Subtract/2
  Switch2/1 -> Switch1/1
  Relational Operator/1 -> Switch3/2
  Subtract1/1 -> Switch3/1
  Constant2/1 -> Subtract1/2
  Min/1 -> Switch3/3, Relational Operator1/2
  Day count/1 -> Relational Operator/2, Switch2/3
  Switch3/1 -> Switch/1
  Function/1 -> Compare To Constant/1
  Switch4/1 -> Output/1
  Compare To Constant/1 -> Switch4/2
  Switch/1 -> Switch4/1
  Down/1 -> Switch1/2
  Up/1 -> Switch/2

== system amg_high_precision_rtc/Soft I2C/Soft-DS3231 Configure/Enabled Subsystem/Subsystem/Enabled Subsystem/Subsystem/Day count ==
  Month : Inport
  Year : Inport  Port=2
  Constant : Constant  Value=30  OutDataTypeStr=uint8
  Constant1 : Constant  Value=31  OutDataTypeStr=uint8
  Days 30 : Subsystem
  Subsystem : Subsystem
  Switch : Switch  Criteria=u2 ~= 0
  Switch1 : Switch  Criteria=u2 ~= 0
  Day count of month : Outport
  wires:
  Switch/1 -> Day count of month/1
  Switch1/1 -> Switch/3
  Constant1/1 -> Switch1/3
  Subsystem/2(Day count) -> Switch1/1
  Subsystem/1(Out1) -> Switch1/2
  Year/1 -> Subsystem/2(Year)
  Month/1 -> Subsystem/1(Month), Days 30/1(In1)
  Constant/1 -> Switch/1
  Days 30/1(Out1) -> Switch/2

== system amg_high_precision_rtc/Soft I2C/Soft-DS3231 Configure/Enabled Subsystem/Subsystem/Enabled Subsystem/Subsystem/Subsystem ==
  Function : Inport
  Input : Inport  Port=2
  Up : Inport  Port=3
  Down : Inport  Port=4
  Day count : Inport  Port=5
  Compare To Constant : simulink/Logic and Bit Operations/Compare To Constant  SystemSampleTime=-1  relop===  const=0  LogicOutDataTypeMode=uint8  ZeroCross=off
  Constant : Constant  OutDataTypeStr=uint8
  Constant2 : Constant  OutDataTypeStr=uint8
  Min : Constant  OutDataTypeStr=uint8
  Relational Operator : RelationalOperator  Operator=<  OutDataTypeStr=boolean
  Relational Operator1 : RelationalOperator  Operator=>  OutDataTypeStr=boolean
  Subtract : Sum  Inputs=+-
  Subtract1 : Sum
  Switch{,1..4} (5 alike) : Switch  Criteria=u2 ~= 0
  Output : Outport
  wires:
  Up/1 -> Switch/2
  Down/1 -> Switch1/2
  Switch/1 -> Switch4/1
  Compare To Constant/1 -> Switch4/2
  Switch4/1 -> Output/1
  Function/1 -> Compare To Constant/1
  Switch3/1 -> Switch/1
  Day count/1 -> Switch2/3, Relational Operator/2
  Min/1 -> Relational Operator1/2, Switch3/3
  Constant2/1 -> Subtract1/2
  Subtract1/1 -> Switch3/1
  Relational Operator/1 -> Switch3/2
  Switch2/1 -> Switch1/1
  Constant/1 -> Subtract/2
  Subtract/1 -> Switch2/1
  Relational Operator1/1 -> Switch2/2
  Input/1 -> Switch4/3, Subtract1/1, Relational Operator/1, Relational Operator1/1, Switch1/3, Subtract/1
  Switch1/1 -> Switch/3

== system amg_high_precision_rtc/Soft I2C/Soft-DS3231 Configure/Enabled Subsystem/Subsystem/Soft-DS3231 Get Date/Convert/Convert 1 ==
  In1 : Inport
  Add : Sum
  Constant : Constant  Value=10  OutDataTypeStr=uint8
  Extract Bits : simulink/Logic and Bit Operations/Extract Bits  SystemSampleTime=-1  bitsToExtract=Range of bits  numBits=8  bitIdxRange=[4 5]  outScalingMode=Treat bit field as an integer
  Extract Bits1 : simulink/Logic and Bit Operations/Extract Bits  SystemSampleTime=-1  bitsToExtract=Range of bits  numBits=8  bitIdxRange=[0 3]  outScalingMode=Treat bit field as an integer
  Product : Product  RndMeth=Zero
  Out1 : Outport
  wires:
  In1/1 -> Extract Bits/1, Extract Bits1/1
  Constant/1 -> Product/1
  Extract Bits/1 -> Product/2
  Product/1 -> Add/1
  Extract Bits1/1 -> Add/2
  Add/1 -> Out1/1

== system amg_high_precision_rtc/Soft I2C/Soft-DS3231 Configure/Enabled Subsystem/Subsystem/Soft-DS3231 Get Date/Convert/Convert 2 ==
  In1 : Inport
  Add : Sum
  Constant : Constant  Value=10  OutDataTypeStr=uint8
  Extract Bits : simulink/Logic and Bit Operations/Extract Bits  SystemSampleTime=-1  bitsToExtract=Range of bits  numBits=8  bitIdxRange=[4 4]  outScalingMode=Treat bit field as an integer
  Extract Bits1 : simulink/Logic and Bit Operations/Extract Bits  SystemSampleTime=-1  bitsToExtract=Range of bits  numBits=8  bitIdxRange=[0 3]  outScalingMode=Treat bit field as an integer
  Product : Product  RndMeth=Zero
  Out1 : Outport
  wires:
  Add/1 -> Out1/1
  Extract Bits1/1 -> Add/2
  Product/1 -> Add/1
  Extract Bits/1 -> Product/2
  Constant/1 -> Product/1
  In1/1 -> Extract Bits1/1, Extract Bits/1

== system amg_high_precision_rtc/Soft I2C/Soft-DS3231 Configure/Enabled Subsystem/Subsystem/Soft-DS3231 Get Date/Convert/Convert 3 ==
  In1 : Inport
  Add : Sum
  Constant : Constant  Value=10  OutDataTypeStr=uint8
  Extract Bits : simulink/Logic and Bit Operations/Extract Bits  SystemSampleTime=-1  bitsToExtract=Range of bits  numBits=8  bitIdxRange=[4 7]  outScalingMode=Treat bit field as an integer
  Extract Bits1 : simulink/Logic and Bit Operations/Extract Bits  SystemSampleTime=-1  bitsToExtract=Range of bits  numBits=8  bitIdxRange=[0 3]  outScalingMode=Treat bit field as an integer
  Product : Product  RndMeth=Zero
  Out1 : Outport
  wires:
  In1/1 -> Extract Bits/1, Extract Bits1/1
  Constant/1 -> Product/1
  Extract Bits/1 -> Product/2
  Product/1 -> Add/1
  Extract Bits1/1 -> Add/2
  Add/1 -> Out1/1

== system amg_high_precision_rtc/Soft I2C/Soft-DS3231 Configure/Enabled Subsystem/Subsystem/Soft-DS3231 Get Time/Convert/Convert Hour ==
  In1 : Inport
  Add : Sum
  Constant : Constant  Value=10  OutDataTypeStr=uint8
  Extract Bits : simulink/Logic and Bit Operations/Extract Bits  SystemSampleTime=-1  bitsToExtract=Range of bits  numBits=8  bitIdxRange=[4 5]  outScalingMode=Treat bit field as an integer
  Extract Bits1 : simulink/Logic and Bit Operations/Extract Bits  SystemSampleTime=-1  bitsToExtract=Range of bits  numBits=8  bitIdxRange=[0 3]  outScalingMode=Treat bit field as an integer
  Extract Bits2 : simulink/Logic and Bit Operations/Extract Bits  SystemSampleTime=-1  bitsToExtract=Range of bits  numBits=8  bitIdxRange=[5 5]  outScalingMode=Treat bit field as an integer
  Product : Product  RndMeth=Zero
  Hour : Outport
  AM/PM : Outport  Port=2
  wires:
  Add/1 -> Hour/1
  Product/1 -> Add/1
  Extract Bits/1 -> Product/2
  Constant/1 -> Product/1
  In1/1 -> Extract Bits/1, Extract Bits1/1, Extract Bits2/1
  Extract Bits1/1 -> Add/2
  Extract Bits2/1 -> AM/PM/1

== system amg_high_precision_rtc/Soft I2C/Soft-DS3231 Configure/Enabled Subsystem/Subsystem/Soft-DS3231 Get Time/Convert/Convert Second// Minute ==
  In1 : Inport
  Add : Sum
  Constant : Constant  Value=10  OutDataTypeStr=uint8
  Extract Bits : simulink/Logic and Bit Operations/Extract Bits  SystemSampleTime=-1  bitsToExtract=Range of bits  numBits=8  bitIdxRange=[4 6]  outScalingMode=Treat bit field as an integer
  Extract Bits1 : simulink/Logic and Bit Operations/Extract Bits  SystemSampleTime=-1  bitsToExtract=Range of bits  numBits=8  bitIdxRange=[0 3]  outScalingMode=Treat bit field as an integer
  Product : Product  RndMeth=Zero
  Out1 : Outport
  wires:
  In1/1 -> Extract Bits/1, Extract Bits1/1
  Constant/1 -> Product/1
  Extract Bits/1 -> Product/2
  Product/1 -> Add/1
  Extract Bits1/1 -> Add/2
  Add/1 -> Out1/1

== system amg_high_precision_rtc/STM32F4/DS3231 Configure/Enabled Subsystem/Subsystem/Enabled Subsystem/Subsystem/Day count/Days 30 ==
  In1 : Inport
  Bitwise Operator : simulink/Logic and Bit Operations/Bitwise Operator  logicop=OR  UseBitMask=off  NumInputPorts=4  BitMask=bin2dec('11011001')  BitMaskRealWorld=Stored Integer
  Compare To Constant : simulink/Logic and Bit Operations/Compare To Constant  SystemSampleTime=-1  relop===  const=6  LogicOutDataTypeMode=uint8  ZeroCross=off
  Compare To Constant1 : simulink/Logic and Bit Operations/Compare To Constant  SystemSampleTime=-1  relop===  const=4  LogicOutDataTypeMode=uint8  ZeroCross=off
  Compare To Constant2 : simulink/Logic and Bit Operations/Compare To Constant  SystemSampleTime=-1  relop===  const=9  LogicOutDataTypeMode=uint8  ZeroCross=off
  Compare To Constant3 : simulink/Logic and Bit Operations/Compare To Constant  SystemSampleTime=-1  relop===  const=11  LogicOutDataTypeMode=uint8  ZeroCross=off
  Out1 : Outport
  wires:
  Compare To Constant1/1 -> Bitwise Operator/1
  Compare To Constant/1 -> Bitwise Operator/2
  Compare To Constant2/1 -> Bitwise Operator/3
  Compare To Constant3/1 -> Bitwise Operator/4
  In1/1 -> Compare To Constant1/1, Compare To Constant/1, Compare To Constant2/1, Compare To Constant3/1
  Bitwise Operator/1 -> Out1/1
